simulink model "Simulation_Model"  (R2023b)
settings: Solver=daessc  StartTime=0.0  StopTime=1  RelTol=1e-3
undefined symbols (not defined in the file): t_sample, X, Y, Z
libraries: sm_lib x7, nesl_utility x1, Simulation_lib x1, SignalEditorBlockLib x1
settings Model: Creator=FIRSTMentor  LastModifiedBy=FIRSTMentor
settings DebuggingCC: UnderspecifiedInitializationDetection=Classic  MergeDetectMultiDrivingBlocksExec=none
settings ModelReferenceCC: PropagateSignalLabelsOutOfModel=off

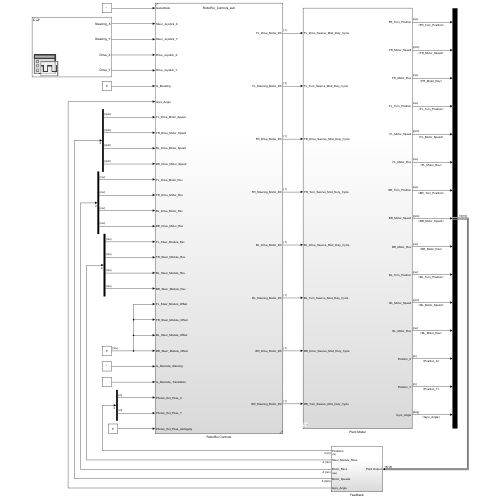
[thumbnail: Simulink's stored preview of the top-level diagram]
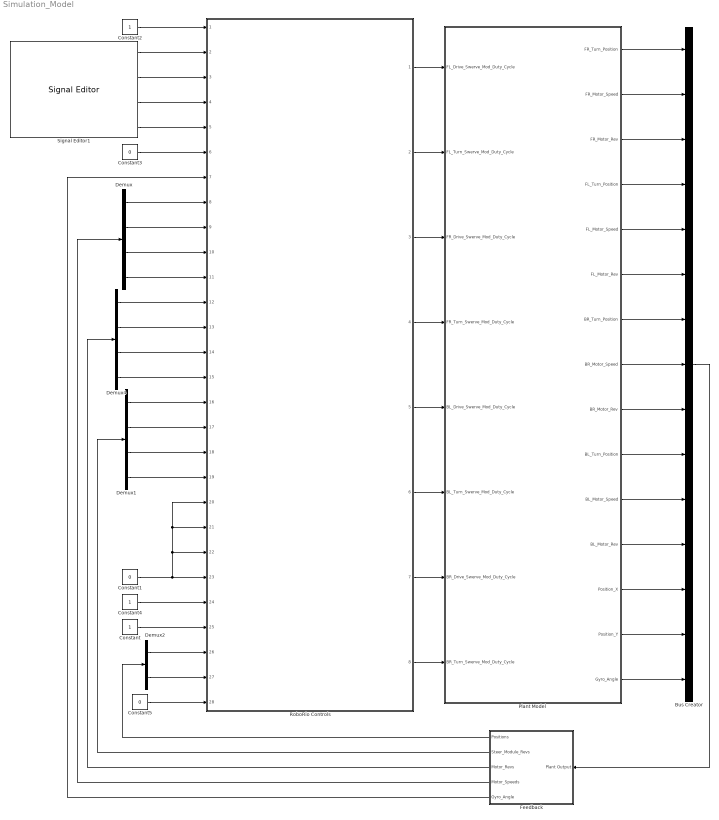
== system Simulation_Model ==
  Bus Creator : BusCreator  Inputs=15
  Constant : Constant  OutDataTypeStr=boolean
  Constant1 : Constant  Value=0
  Constant2 : Constant
  Constant3 : Constant  Value=0  OutDataTypeStr=boolean
  Constant4 : Constant  OutDataTypeStr=boolean
  Constant5 : Constant  Value=0  OutDataTypeStr=double
  Demux : Demux
  Demux1 : Demux
  Demux2 : Demux  Outputs=2
  Demux4 : Demux
  Feedback : Subsystem
  Plant Model : Subsystem  AncestorBlock=Simulation_lib/Simulation_Top
  RoboRio Controls : Subsystem  ReferencedSubsystem=RoboRio_Controls_sub
  Signal Editor1 : SignalEditorBlockLib/Signal Editor  FileName=Joystick_input_test_data.mat  ActiveScenario=DXP  ActiveSignal=Drive_Y  IsBus=off  OutputBusObjectStr=Bus: BusObject  SampleTime=t_sample  ZeroCross=off  OutputAfterFinalValue=Setting to zero  Unit=inherit  PreserveSignalName=on  ApplySigPropsToAllScenarios=on  ApplySigPropsToAllSignals=off
  wires:
  RoboRio Controls/3 -> Plant Model/3(FR_Drive_Swerve_Mod_Duty_Cycle)
  RoboRio Controls/2 -> Plant Model/2(FL_Turn_Swerve_Mod_Duty_Cycle)
  RoboRio Controls/4 -> Plant Model/4(FR_Turn_Swerve_Mod_Duty_Cycle)
  RoboRio Controls/1 -> Plant Model/1(FL_Drive_Swerve_Mod_Duty_Cycle)
  RoboRio Controls/5 -> Plant Model/5(BL_Drive_Swerve_Mod_Duty_Cycle)
  RoboRio Controls/6 -> Plant Model/6(BL_Turn_Swerve_Mod_Duty_Cycle)
  RoboRio Controls/7 -> Plant Model/7(BR_Drive_Swerve_Mod_Duty_Cycle)
  RoboRio Controls/8 -> Plant Model/8(BR_Turn_Swerve_Mod_Duty_Cycle)
  Constant/1 -> RoboRio Controls/25
  Constant1/1 -> RoboRio Controls/20, RoboRio Controls/21, RoboRio Controls/22, RoboRio Controls/23
  Constant2/1 -> RoboRio Controls/1
  Signal Editor1/2 -> RoboRio Controls/3
  Signal Editor1/4 -> RoboRio Controls/5
  Constant3/1 -> RoboRio Controls/6
  Signal Editor1/3 -> RoboRio Controls/4
  Signal Editor1/1 -> RoboRio Controls/2
  Constant4/1 -> RoboRio Controls/24
  Plant Model/7(BR_Turn_Position) -> Bus Creator/7
  Plant Model/6(FL_Motor_Rev) -> Bus Creator/6
  Plant Model/8(BR_Motor_Speed) -> Bus Creator/8
  Plant Model/5(FL_Motor_Speed) -> Bus Creator/5
  Plant Model/9(BR_Motor_Rev) -> Bus Creator/9
  Plant Model/4(FL_Turn_Position) -> Bus Creator/4
  Plant Model/10(BL_Turn_Position) -> Bus Creator/10
  Plant Model/3(FR_Motor_Rev) -> Bus Creator/3
  Plant Model/11(BL_Motor_Speed) -> Bus Creator/11
  Plant Model/2(FR_Motor_Speed) -> Bus Creator/2
  Plant Model/12(BL_Motor_Rev) -> Bus Creator/12
  Plant Model/1(FR_Turn_Position) -> Bus Creator/1
  Plant Model/13(Position_X) -> Bus Creator/13
  Bus Creator/1 -> Feedback/1(Plant Output)
  Feedback/4(Motor_Speeds) -> Demux/1
  Demux/2 -> RoboRio Controls/9
  Demux/1 -> RoboRio Controls/8
  Demux/3 -> RoboRio Controls/10
  Demux/4 -> RoboRio Controls/11
  Demux1/1 -> RoboRio Controls/16
  Demux1/2 -> RoboRio Controls/17
  Demux1/3 -> RoboRio Controls/18
  Demux1/4 -> RoboRio Controls/19
  Feedback/2(Steer_Module_Revs) -> Demux1/1
  Feedback/5(Gyro_Angle) -> RoboRio Controls/7
  Demux4/1 -> RoboRio Controls/12
  Demux4/2 -> RoboRio Controls/13
  Demux4/3 -> RoboRio Controls/14
  Demux4/4 -> RoboRio Controls/15
  Feedback/3(Motor_Revs) -> Demux4/1
  Plant Model/14(Position_Y) -> Bus Creator/14
  Plant Model/15(Gyro_Angle) -> Bus Creator/15
  Demux2/2 -> RoboRio Controls/27
  Demux2/1 -> RoboRio Controls/26
  Feedback/1(Positions) -> Demux2/1
  Constant5/1 -> RoboRio Controls/28

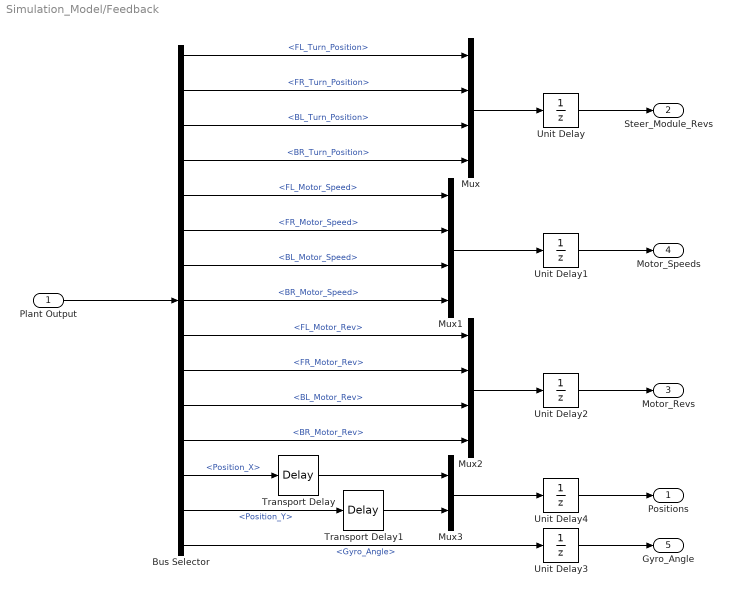
== system Simulation_Model/Feedback ==
  Plant Output : Inport
  Bus Selector : BusSelector  OutputSignals=FL_Turn_Position,FR_Turn_Position,BL_Turn_Position,BR_Turn_Position,FL_Motor_Speed,FR_Motor_Speed,BL_Motor_Speed,BR_Motor_Speed,FL_Motor_Rev,FR_Motor_Rev,BL_Motor_Rev,BR_Motor_Rev,Position_X,Position_Y,Gyro_Angle
  Mux : Mux
  Mux1 : Mux
  Mux2 : Mux
  Mux3 : Mux  Inputs=2
  Transport Delay : TransportDelay  DelayTime=0.12
  Transport Delay1 : TransportDelay  DelayTime=0.12
  Unit Delay : UnitDelay  InitialCondition=[0 0 0 0]  SampleTime=t_sample  HasFrameUpgradeWarning=on
  Unit Delay1 : UnitDelay  InitialCondition=[0 0 0 0]  SampleTime=t_sample  HasFrameUpgradeWarning=on
  Unit Delay2 : UnitDelay  InitialCondition=[0 0 0 0]  SampleTime=t_sample  HasFrameUpgradeWarning=on
  Unit Delay3 : UnitDelay  SampleTime=t_sample  HasFrameUpgradeWarning=on
  Unit Delay4 : UnitDelay  SampleTime=t_sample  HasFrameUpgradeWarning=on
  Positions : Outport  Unit=m
  Steer_Module_Revs : Outport  Port=2
  Motor_Revs : Outport  Port=3  Unit=rev
  Motor_Speeds : Outport  Port=4
  Gyro_Angle : Outport  Port=5
  wires:
  Plant Output/1 -> Bus Selector/1
  Mux/1 -> Unit Delay/1
  Mux1/1 -> Unit Delay1/1
  Mux2/1 -> Unit Delay2/1
  Bus Selector/15 -> Unit Delay3/1  "<Gyro_Angle>"
  Bus Selector/1 -> Mux/1  "<FL_Turn_Position>"
  Bus Selector/2 -> Mux/2  "<FR_Turn_Position>"
  Bus Selector/3 -> Mux/3  "<BL_Turn_Position>"
  Bus Selector/4 -> Mux/4  "<BR_Turn_Position>"
  Bus Selector/5 -> Mux1/1  "<FL_Motor_Speed>"
  Bus Selector/6 -> Mux1/2  "<FR_Motor_Speed>"
  Bus Selector/7 -> Mux1/3  "<BL_Motor_Speed>"
  Bus Selector/8 -> Mux1/4  "<BR_Motor_Speed>"
  Bus Selector/9 -> Mux2/1  "<FL_Motor_Rev>"
  Bus Selector/10 -> Mux2/2  "<FR_Motor_Rev>"
  Bus Selector/11 -> Mux2/3  "<BL_Motor_Rev>"
  Bus Selector/12 -> Mux2/4  "<BR_Motor_Rev>"
  Unit Delay/1 -> Steer_Module_Revs/1
  Unit Delay1/1 -> Motor_Speeds/1
  Unit Delay2/1 -> Motor_Revs/1
  Unit Delay3/1 -> Gyro_Angle/1
  Bus Selector/13 -> Transport Delay/1  "<Position_X>"
  Bus Selector/14 -> Transport Delay1/1  "<Position_Y>"
  Mux3/1 -> Unit Delay4/1
  Unit Delay4/1 -> Positions/1
  Transport Delay/1 -> Mux3/1
  Transport Delay1/1 -> Mux3/2

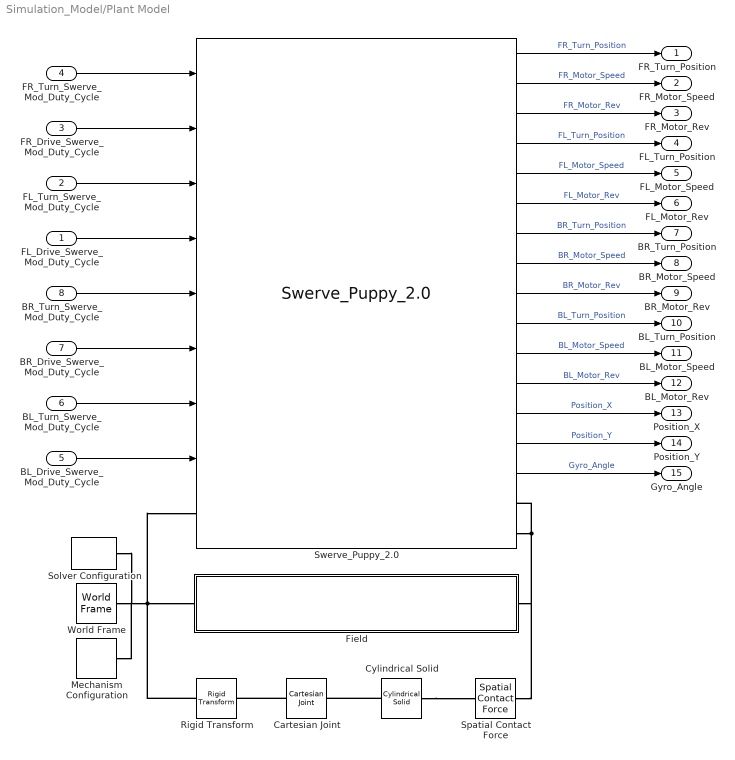
== system Simulation_Model/Plant Model ==
  FL_Drive_Swerve_Mod_Duty_Cycle : Inport
  FL_Turn_Swerve_Mod_Duty_Cycle : Inport  Port=2
  FR_Drive_Swerve_Mod_Duty_Cycle : Inport  Port=3
  FR_Turn_Swerve_Mod_Duty_Cycle : Inport  Port=4
  BL_Drive_Swerve_Mod_Duty_Cycle : Inport  Port=5
  BL_Turn_Swerve_Mod_Duty_Cycle : Inport  Port=6
  BR_Drive_Swerve_Mod_Duty_Cycle : Inport  Port=7
  BR_Turn_Swerve_Mod_Duty_Cycle : Inport  Port=8
  Cartesian Joint : sm_lib/Joints/Cartesian Joint  JointMode=Normal  SenseConstraintForce=off  SenseConstraintForceX=off  SenseConstraintForceY=off  SenseConstraintForceZ=off  SenseConstraintTorque=off  SenseConstraintTorqueX=off  SenseConstraintTorqueY=off  SenseConstraintTorqueZ=off  SenseTotalForce=off  SenseTotalForceX=off  SenseTotalForceY=off  SenseTotalForceZ=off  SenseTotalTorque=off  SenseTotalTorqueX=off  SenseTotalTorqueY=off  SenseTotalTorqueZ=off  CompositeWrenchDir=FollowerOnBase  CompositeWrenchFrame=BaseFrame  PxEquilibriumPosition=0  PxEquilibriumPositionUnits=m  PxSpringStiffness=0  PxSpringStiffnessUnits=N/m  PxDampingCoefficient=0  PxDampingCoefficientUnits=N/(m/s)  PxTorqueActuationMode=NoTorque  PxMotionActuationMode=ComputedMotion  PxSensePosition=off  PxSenseVelocity=off  PxSenseAcceleration=off  PxSenseTorqueForce=off  PxSenseLowerLimitTorqueForce=off  PxSenseUpperLimitTorqueForce=off  PxLowerLimitSpecify=off  PxLowerLimitBound=-1  PxLowerLimitBoundUnits=m  PxLowerLimitStiffness=1e6  PxLowerLimitStiffnessUnits=N/m  PxLowerLimitDamping=1e3  PxLowerLimitDampingUnits=N/(m/s)  PxLowerLimitTransitionRegionWidth=1e-4  PxLowerLimitTransitionRegionWidthUnits=m  PxUpperLimitSpecify=off  PxUpperLimitBound=1  PxUpperLimitBoundUnits=m  PxUpperLimitStiffness=1e6  PxUpperLimitStiffnessUnits=N/m  PxUpperLimitDamping=1e3  PxUpperLimitDampingUnits=N/(m/s)  PxUpperLimitTransitionRegionWidth=1e-4  PxUpperLimitTransitionRegionWidthUnits=m  PxPositionTargetSpecify=off  PxPositionTargetPriority=High  PxPositionTargetValue=0  PxPositionTargetValueUnits=m  PxVelocityTargetSpecify=off  PxVelocityTargetPriority=High  PxVelocityTargetValue=0  PxVelocityTargetValueUnits=m/s  PyEquilibriumPosition=0  PyEquilibriumPositionUnits=m  PySpringStiffness=0  PySpringStiffnessUnits=N/m  PyDampingCoefficient=0  PyDampingCoefficientUnits=N/(m/s)  PyTorqueActuationMode=NoTorque  PyMotionActuationMode=ComputedMotion  PySensePosition=off  PySenseVelocity=off  PySenseAcceleration=off  PySenseTorqueForce=off  PySenseLowerLimitTorqueForce=off  PySenseUpperLimitTorqueForce=off  PyLowerLimitSpecify=off  PyLowerLimitBound=-1  PyLowerLimitBoundUnits=m  PyLowerLimitStiffness=1e6  PyLowerLimitStiffnessUnits=N/m  PyLowerLimitDamping=1e3  PyLowerLimitDampingUnits=N/(m/s)  PyLowerLimitTransitionRegionWidth=1e-4  PyLowerLimitTransitionRegionWidthUnits=m  PyUpperLimitSpecify=off  PyUpperLimitBound=1  PyUpperLimitBoundUnits=m  PyUpperLimitStiffness=1e6  PyUpperLimitStiffnessUnits=N/m  PyUpperLimitDamping=1e3  PyUpperLimitDampingUnits=N/(m/s)  PyUpperLimitTransitionRegionWidth=1e-4  PyUpperLimitTransitionRegionWidthUnits=m  PyPositionTargetSpecify=off  PyPositionTargetPriority=High  PyPositionTargetValue=0  PyPositionTargetValueUnits=m  PyVelocityTargetSpecify=off  PyVelocityTargetPriority=High  PyVelocityTargetValue=0  PyVelocityTargetValueUnits=m/s  PzEquilibriumPosition=0  PzEquilibriumPositionUnits=m  PzSpringStiffness=0  PzSpringStiffnessUnits=N/m  PzDampingCoefficient=0  PzDampingCoefficientUnits=N/(m/s)  PzTorqueActuationMode=NoTorque  PzMotionActuationMode=ComputedMotion  PzSensePosition=off  PzSenseVelocity=off  PzSenseAcceleration=off  PzSenseTorqueForce=off  PzSenseLowerLimitTorqueForce=off  PzSenseUpperLimitTorqueForce=off  PzLowerLimitSpecify=off  PzLowerLimitBound=-1  PzLowerLimitBoundUnits=m  PzLowerLimitStiffness=1e6  PzLowerLimitStiffnessUnits=N/m  PzLowerLimitDamping=1e3  PzLowerLimitDampingUnits=N/(m/s)  PzLowerLimitTransitionRegionWidth=1e-4  PzLowerLimitTransitionRegionWidthUnits=m  PzUpperLimitSpecify=off  PzUpperLimitBound=1  PzUpperLimitBoundUnits=m  PzUpperLimitStiffness=1e6  PzUpperLimitStiffnessUnits=N/m  PzUpperLimitDamping=1e3  PzUpperLimitDampingUnits=N/(m/s)  PzUpperLimitTransitionRegionWidth=1e-4  PzUpperLimitTransitionRegionWidthUnits=m  PzPositionTargetSpecify=off  PzPositionTargetPriority=High  PzPositionTargetValue=0  PzPositionTargetValueUnits=m  PzVelocityTargetSpecify=off  PzVelocityTargetPriority=High  PzVelocityTargetValue=0  PzVelocityTargetValueUnits=m/s
  Cylindrical Solid : sm_lib/Body Elements/Cylindrical Solid  GraphicAmbientColor=[0.15 0.15 0.15 1.0]  BasedOnType=Density  CenterOfMass=[0 0 0]  CenterOfMassUnits=m  GraphicDiffuseColor=[0.5 0.5 0.5]  CylinderLength=2  CylinderLengthUnits=in  CylinderRadius=7  CylinderRadiusUnits=in  Density=1000  DensityUnits=kg/m^3  DoExposeReferenceFrame=on  GraphicEmissiveColor=[0.0 0.0 0.0 1.0]  ExportEntireGeometry=on  SerializedFrames=<Frames/>  MarkerShape=Sphere  MarkerSize=10  GraphicType=FromGeometry  InertiaType=CalculateFromGeometry  Mass=1  MassUnits=kg  MomentsOfInertia=[1 1 1]  MomentsOfInertiaUnits=kg*m^2  GraphicOpacity=1.0  ProductsOfInertia=[0 0 0]  ProductsOfInertiaUnits=kg*m^2  GraphicShininess=75  GraphicSpecularColor=[0.5 0.5 0.5 1.0]  GraphicVisPropType=SimpleVisualProperties
  Field : Subsystem  AncestorBlock=Simulation_lib/Field
  Mechanism Configuration : sm_lib/Utilities/Mechanism Configuration  UniformGravity=Constant  GravityVector=[0 0 -9.80665]  GravityVectorUnits=m/s^2  LinearizationDelta=0.001  JointModeTransitionNonlinearIterations=2
  Rigid Transform : sm_lib/Frames and Transforms/Rigid Transform  TranslationMethod=StandardAxis  TranslationStandardOffset=1  TranslationStandardOffsetUnits=m  TranslationStandardAxis=+Z  TranslationCartesianOffset=[0 0 0]  TranslationCartesianOffsetUnits=m  TranslationROffset=0  TranslationROffsetUnits=m  TranslationZOffset=0  TranslationZOffsetUnits=m  TranslationThetaOffset=0  TranslationThetaOffsetUnits=deg  RotationMethod=None  RotationAngleUnits=deg  RotationStandardAxis=+Z  RotationAngle=2  RotationArbitraryAxis=[0 0 1]  FollAlignAxisA=+X  BaseAlignAxisA=+Y  FollAlignAxisB=+Y  BaseAlignAxisB=+Z  RotationSequenceAxes=FollowerAxes  RotationSequence=XYX  RotationSequenceAngles=[0 0 0]  RotationSequenceAnglesUnits=deg  RotationMatrix=[1 0 0; 0 1 0; 0 0 1]  Quaternion=[1 0 0 0]
  Solver Configuration : nesl_utility/Solver Configuration  PhysicalDomain=network_engine_domain  SubClassName=solver  LeftPortType=input  RightPortType=generic  Tones=[]  Harmonics=[]  SimulateNoise=off  Profile=off  UseLocalSampling=off  EnableSwitchedLinearOptims=on  FrequencyDomain=off  UseCCode=off  RelTol=0.001  AbsTol=0.001  MinStep=1e-09  ToWorkspace=off  RevertToSquareIcSolve=off  NumHomotopyIterations=100  PhasorMode=off  PhasorModeNumHarmonics=1  ConsistencySolver=NEWTON_XTOL_AFTER_FTOL  IndexReductionMethod=DerivativeReplacement  DoDC=off  ResidualTolerance=1e-09  ConsistencyTolSource=GLOBAL  ConsistencyAbsTol=0.001  ConsistencyRelTol=0.001  ConsistencyTolFactor=0.001  UseLocalSolver=off  LocalSolverChoice=NE_BACKWARD_EULER_ADVANCER  ResolveIndetEquations=on  FunctionEvalNumThread=1  LocalSolverSampleTime=0.001  DoFixedCost=off  MaxNonlinIter=3  MaxModeIter=2  ComputeImpulses=off  ImpulseIterations=2  LinearAlgebra=auto  LinearAlgebraNumThread=0  EquationFormulation=NE_TIME_EF  DelaysMemoryBudget=1024  AutomaticFiltering=on  FilteringTimeConstant=0.001  PartitionStorageMethod=AS_NEEDED  PartitionMemoryBudget=1024  PartitionMethod=ROBUST  MultibodyUseLocalSolver=off  MultibodyLocalSolverChoice=ODE1  MultibodyLocalSolverSampleTime=0.001
  Spatial Contact Force : sm_lib/Forces and Torques/Spatial Contact Force  SenseContactBaseRotation=off  SenseContactBaseTranslation=off  CoefficientOfDynamicFriction=0.3  CoefficientOfStaticFriction=0.5  NormalDamping=1e3  NormalDampingUnits=N/(m/s)  SenseContactSignal=off  NormalStiffness=1e6  NormalStiffnessUnits=N/m  FrictionalCriticalVelocity=1e-3  FrictionalCriticalVelocityUnits=m/s  ZeroCrossDetectContactStartAndEnd=off  SenseContactFollowerRotation=off  SenseContactFollowerTranslation=off  FrictionType=SmoothStickSlip  SenseFrictionalForceMagnitude=off  SenseNormalForceMagnitude=off  NormalForceType=SmoothSpringDamper  SenseNormalVelocity=off  SensePenetrationDepth=off  SenseSeparationDistance=off  SenseTangentialVelocity=off  NormalTransitionRegionWidth=1e-4  NormalTransitionRegionWidthUnits=m
  Swerve_Puppy_2.0 : Simulation_lib/Swerve_Puppy_2.0  SystemSampleTime=-1  VariantActivationTime=update diagram  AllowFlexibleInterface=on  Latency=0  AutoFrameSizeCalculation=off
  World Frame : sm_lib/Frames and Transforms/World Frame
  FR_Turn_Position : Outport
  FR_Motor_Speed : Outport  Port=2
  FR_Motor_Rev : Outport  Port=3
  FL_Turn_Position : Outport  Port=4
  FL_Motor_Speed : Outport  Port=5
  FL_Motor_Rev : Outport  Port=6
  BR_Turn_Position : Outport  Port=7
  BR_Motor_Speed : Outport  Port=8
  BR_Motor_Rev : Outport  Port=9
  BL_Turn_Position : Outport  Port=10
  BL_Motor_Speed : Outport  Port=11
  BL_Motor_Rev : Outport  Port=12
  Position_X : Outport  Port=13
  Position_Y : Outport  Port=14
  Gyro_Angle : Outport  Port=15
  wires:
  Swerve_Puppy_2.0/14 -> Position_Y/1  "Position_Y"
  Swerve_Puppy_2.0/13 -> Position_X/1  "Position_X"
  Swerve_Puppy_2.0/12 -> BL_Motor_Rev/1  "BL_Motor_Rev"
  Swerve_Puppy_2.0/9 -> BR_Motor_Rev/1  "BR_Motor_Rev"
  Swerve_Puppy_2.0/6 -> FL_Motor_Rev/1  "FL_Motor_Rev"
  Swerve_Puppy_2.0/3 -> FR_Motor_Rev/1  "FR_Motor_Rev"
  Swerve_Puppy_2.0/11 -> BL_Motor_Speed/1  "BL_Motor_Speed"
  Swerve_Puppy_2.0/10 -> BL_Turn_Position/1  "BL_Turn_Position"
  Swerve_Puppy_2.0/8 -> BR_Motor_Speed/1  "BR_Motor_Speed"
  Swerve_Puppy_2.0/7 -> BR_Turn_Position/1  "BR_Turn_Position"
  Swerve_Puppy_2.0/5 -> FL_Motor_Speed/1  "FL_Motor_Speed"
  Swerve_Puppy_2.0/4 -> FL_Turn_Position/1  "FL_Turn_Position"
  Swerve_Puppy_2.0/2 -> FR_Motor_Speed/1  "FR_Motor_Speed"
  Swerve_Puppy_2.0/1 -> FR_Turn_Position/1  "FR_Turn_Position"
  Swerve_Puppy_2.0/15 -> Gyro_Angle/1  "Gyro_Angle"
  BL_Drive_Swerve_Mod_Duty_Cycle/1 -> Swerve_Puppy_2.0/8
  BL_Turn_Swerve_Mod_Duty_Cycle/1 -> Swerve_Puppy_2.0/7
  BR_Drive_Swerve_Mod_Duty_Cycle/1 -> Swerve_Puppy_2.0/6
  BR_Turn_Swerve_Mod_Duty_Cycle/1 -> Swerve_Puppy_2.0/5
  FL_Drive_Swerve_Mod_Duty_Cycle/1 -> Swerve_Puppy_2.0/4
  FL_Turn_Swerve_Mod_Duty_Cycle/1 -> Swerve_Puppy_2.0/3
  FR_Drive_Swerve_Mod_Duty_Cycle/1 -> Swerve_Puppy_2.0/2
  FR_Turn_Swerve_Mod_Duty_Cycle/1 -> Swerve_Puppy_2.0/1
  connections:
  Cartesian Joint/LConn1 -- Rigid Transform/RConn1
  Cylindrical Solid/RConn1 -- Cartesian Joint/RConn1
  Spatial Contact Force/RConn1 -- Field/RConn1 -- Swerve_Puppy_2.0/RConn1 -- Swerve_Puppy_2.0/RConn2
  Rigid Transform/LConn1 -- Field/LConn1 -- Swerve_Puppy_2.0/LConn1 -- Solver Configuration/RConn1 -- Mechanism Configuration/RConn1 -- World Frame/RConn1
  Cylindrical Solid/LConn1 -- Spatial Contact Force/LConn1

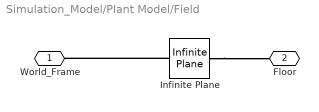
== system Simulation_Model/Plant Model/Field ==
  Infinite Plane : sm_lib/Curves and Surfaces/Infinite Plane  GraphicType=Rectangle  GraphicPlaneWidth=10  GraphicPlaneWidthUnits=m  GraphicPlaneHeight=10  GraphicPlaneHeightUnits=m  GraphicVisPropType=SimpleVisualProperties  GraphicDiffuseColor=[1 0.4118 0.1608]  GraphicOpacity=0.25  GraphicSpecularColor=[0.5 0.5 0.5 1.0]  GraphicAmbientColor=[0.15 0.15 0.15 1.0]  GraphicEmissiveColor=[0.0 0.0 0.0 1.0]  GraphicShininess=75
  World_Frame : PMIOPort  Side=Left
  Floor : PMIOPort  Port=2  Side=Right
  connections:
  Infinite Plane/RConn1 -- Floor/RConn1
  Infinite Plane/LConn1 -- World_Frame/RConn1
